simulink model "AECambioModoAutMan"  (R2020b)
settings: Solver=VariableStepAuto  StartTime=0.0  StopTime=50  RelTol=1e-3
settings Model: Creator=Juan  LastModifiedBy=Juan

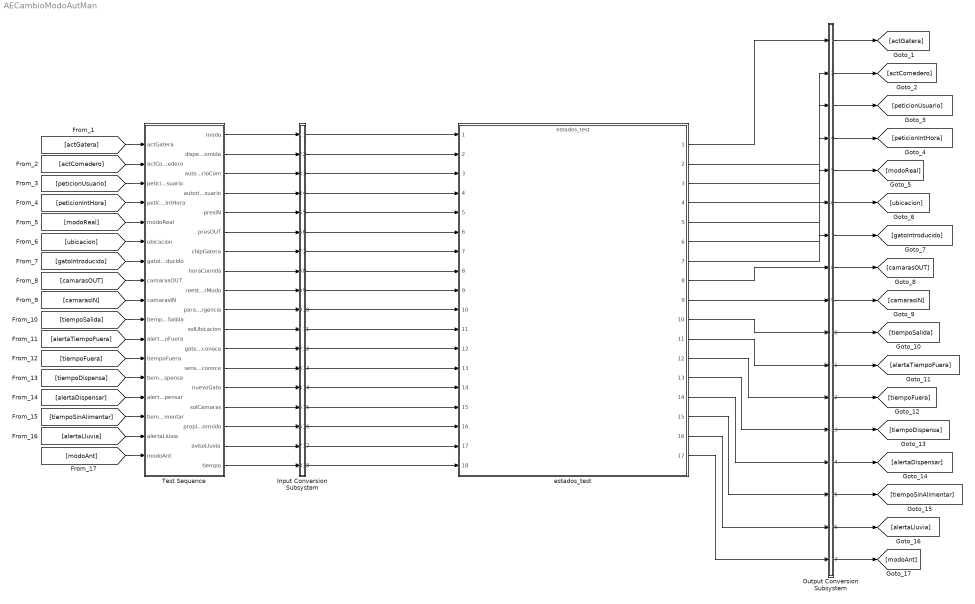
== system AECambioModoAutMan ==
  Input Conversion Subsystem : Subsystem  Tag=__SLT_ICS__  Description=|
      | Signal spec.
      | and routing
      settings: AttributesFormatString=%<Description>
  Output Conversion Subsystem : Subsystem  Tag=__SLT_OCS__  Description=|
      | Signal spec.
      | and routing
      settings: AttributesFormatString=%<Description>
  Test Sequence : Test Sequence  TreatAsAtomicUnit=on
  estados_test : ModelReference  ModelNameDialog=estados_test  SimulationMode=Normal  ModelReferenceVersion=2.162
  wires:
  Test Sequence/1(modo) -> Input Conversion Subsystem/1(Inport_1)
  Test Sequence/2(dispensaComida) -> Input Conversion Subsystem/2(Inport_2)
  Test Sequence/3(autorizUsuarioCom) -> Input Conversion Subsystem/3(Inport_3)
  Test Sequence/4(autorizUsuario) -> Input Conversion Subsystem/4(Inport_4)
  Test Sequence/5(presIN) -> Input Conversion Subsystem/5(Inport_5)
  Test Sequence/6(presOUT) -> Input Conversion Subsystem/6(Inport_6)
  Test Sequence/7(chipGatera) -> Input Conversion Subsystem/7(Inport_7)
  Test Sequence/8(horaComida) -> Input Conversion Subsystem/8(Inport_8)
  Test Sequence/9(reestablecerModo) -> Input Conversion Subsystem/9(Inport_9)
  Test Sequence/10(paradaEmergencia) -> Input Conversion Subsystem/10(Inport_10)
  Test Sequence/11(solUbicacion) -> Input Conversion Subsystem/11(Inport_11)
  Test Sequence/12(gateraReconoce) -> Input Conversion Subsystem/12(Inport_12)
  Test Sequence/13(sensorReconoce) -> Input Conversion Subsystem/13(Inport_13)
  Test Sequence/14(nuevoGato) -> Input Conversion Subsystem/14(Inport_14)
  Test Sequence/15(solCamaras) -> Input Conversion Subsystem/15(Inport_15)
  Test Sequence/16(propietarioDormido) -> Input Conversion Subsystem/16(Inport_16)
  Test Sequence/17(avisoLluvia) -> Input Conversion Subsystem/17(Inport_17)
  Test Sequence/18(tiempo) -> Input Conversion Subsystem/18(Inport_18)
  [actGatera] -> Test Sequence/1(actGatera)
  [actComedero] -> Test Sequence/2(actComedero)
  [peticionUsuario] -> Test Sequence/3(peticionUsuario)
  [peticionIntHora] -> Test Sequence/4(peticionIntHora)
  [modoReal] -> Test Sequence/5(modoReal)
  [ubicacion] -> Test Sequence/6(ubicacion)
  [gatoIntroducido] -> Test Sequence/7(gatoIntroducido)
  [camarasOUT] -> Test Sequence/8(camarasOUT)
  [camarasIN] -> Test Sequence/9(camarasIN)
  [tiempoSalida] -> Test Sequence/10(tiempoSalida)
  [alertaTiempoFuera] -> Test Sequence/11(alertaTiempoFuera)
  [tiempoFuera] -> Test Sequence/12(tiempoFuera)
  [tiempoDispensa] -> Test Sequence/13(tiempoDispensa)
  [alertaDispensar] -> Test Sequence/14(alertaDispensar)
  [tiempoSinAlimentar] -> Test Sequence/15(tiempoSinAlimentar)
  [alertaLluvia] -> Test Sequence/16(alertaLluvia)
  [modoAnt] -> Test Sequence/17(modoAnt)
  Output Conversion Subsystem/1(Outport_1) -> [actGatera]
  Output Conversion Subsystem/2(Outport_2) -> [actComedero]
  Output Conversion Subsystem/3(Outport_3) -> [peticionUsuario]
  Output Conversion Subsystem/4(Outport_4) -> [peticionIntHora]
  Output Conversion Subsystem/5(Outport_5) -> [modoReal]
  Output Conversion Subsystem/6(Outport_6) -> [ubicacion]
  Output Conversion Subsystem/7(Outport_7) -> [gatoIntroducido]
  Output Conversion Subsystem/8(Outport_8) -> [camarasOUT]
  Output Conversion Subsystem/9(Outport_9) -> [camarasIN]
  Output Conversion Subsystem/10(Outport_10) -> [tiempoSalida]
  Output Conversion Subsystem/11(Outport_11) -> [alertaTiempoFuera]
  Output Conversion Subsystem/12(Outport_12) -> [tiempoFuera]
  Output Conversion Subsystem/13(Outport_13) -> [tiempoDispensa]
  Output Conversion Subsystem/14(Outport_14) -> [alertaDispensar]
  Output Conversion Subsystem/15(Outport_15) -> [tiempoSinAlimentar]
  Output Conversion Subsystem/16(Outport_16) -> [alertaLluvia]
  Output Conversion Subsystem/17(Outport_17) -> [modoAnt]
  Input Conversion Subsystem/1(Outport_1) -> estados_test/1
  Input Conversion Subsystem/2(Outport_2) -> estados_test/2
  Input Conversion Subsystem/3(Outport_3) -> estados_test/3
  Input Conversion Subsystem/4(Outport_4) -> estados_test/4
  Input Conversion Subsystem/5(Outport_5) -> estados_test/5
  Input Conversion Subsystem/6(Outport_6) -> estados_test/6
  Input Conversion Subsystem/7(Outport_7) -> estados_test/7
  Input Conversion Subsystem/8(Outport_8) -> estados_test/8
  Input Conversion Subsystem/9(Outport_9) -> estados_test/9
  Input Conversion Subsystem/10(Outport_10) -> estados_test/10
  Input Conversion Subsystem/11(Outport_11) -> estados_test/11
  Input Conversion Subsystem/12(Outport_12) -> estados_test/12
  Input Conversion Subsystem/13(Outport_13) -> estados_test/13
  Input Conversion Subsystem/14(Outport_14) -> estados_test/14
  Input Conversion Subsystem/15(Outport_15) -> estados_test/15
  Input Conversion Subsystem/16(Outport_16) -> estados_test/16
  Input Conversion Subsystem/17(Outport_17) -> estados_test/17
  Input Conversion Subsystem/18(Outport_18) -> estados_test/18
  estados_test/1 -> Output Conversion Subsystem/1(Inport_1)
  estados_test/2 -> Output Conversion Subsystem/2(Inport_2)
  estados_test/3 -> Output Conversion Subsystem/3(Inport_3)
  estados_test/4 -> Output Conversion Subsystem/4(Inport_4)
  estados_test/5 -> Output Conversion Subsystem/5(Inport_5)
  estados_test/6 -> Output Conversion Subsystem/6(Inport_6)
  estados_test/7 -> Output Conversion Subsystem/7(Inport_7)
  estados_test/8 -> Output Conversion Subsystem/8(Inport_8)
  estados_test/9 -> Output Conversion Subsystem/9(Inport_9)
  estados_test/10 -> Output Conversion Subsystem/10(Inport_10)
  estados_test/11 -> Output Conversion Subsystem/11(Inport_11)
  estados_test/12 -> Output Conversion Subsystem/12(Inport_12)
  estados_test/13 -> Output Conversion Subsystem/13(Inport_13)
  estados_test/14 -> Output Conversion Subsystem/14(Inport_14)
  estados_test/15 -> Output Conversion Subsystem/15(Inport_15)
  estados_test/16 -> Output Conversion Subsystem/16(Inport_16)
  estados_test/17 -> Output Conversion Subsystem/17(Inport_17)

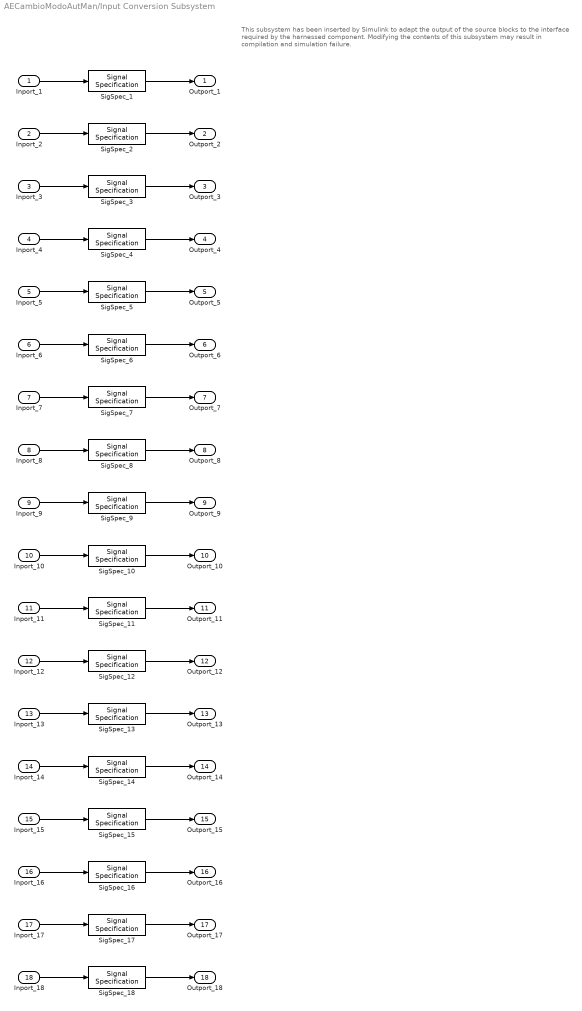
== system AECambioModoAutMan/Input Conversion Subsystem ==
  note: This subsystem has been inserted by Simulink to adapt the output of the source blocks to the interface required by the harnessed component.
      |  Modifying the contents of this subsystem may result in compilation and simulation failure.
  Inport_1 : Inport
  Inport_2 : Inport  Port=2
  Inport_3 : Inport  Port=3
  Inport_4 : Inport  Port=4
  Inport_5 : Inport  Port=5
  Inport_6 : Inport  Port=6
  Inport_7 : Inport  Port=7
  Inport_8 : Inport  Port=8
  Inport_9 : Inport  Port=9
  Inport_10 : Inport  Port=10
  Inport_11 : Inport  Port=11
  Inport_12 : Inport  Port=12
  Inport_13 : Inport  Port=13
  Inport_14 : Inport  Port=14
  Inport_15 : Inport  Port=15
  Inport_16 : Inport  Port=16
  Inport_17 : Inport  Port=17
  Inport_18 : Inport  Port=18
  SigSpec_{1..18} (18 alike) : SignalSpecification  OutDataTypeStr=double  Dimensions=[1]  SampleTime=[-1, 0]
  Outport_1 : Outport
  Outport_2 : Outport  Port=2
  Outport_3 : Outport  Port=3
  Outport_4 : Outport  Port=4
  Outport_5 : Outport  Port=5
  Outport_6 : Outport  Port=6
  Outport_7 : Outport  Port=7
  Outport_8 : Outport  Port=8
  Outport_9 : Outport  Port=9
  Outport_10 : Outport  Port=10
  Outport_11 : Outport  Port=11
  Outport_12 : Outport  Port=12
  Outport_13 : Outport  Port=13
  Outport_14 : Outport  Port=14
  Outport_15 : Outport  Port=15
  Outport_16 : Outport  Port=16
  Outport_17 : Outport  Port=17
  Outport_18 : Outport  Port=18
  wires:
  SigSpec_1/1 -> Outport_1/1
  Inport_1/1 -> SigSpec_1/1
  SigSpec_2/1 -> Outport_2/1
  Inport_2/1 -> SigSpec_2/1
  SigSpec_3/1 -> Outport_3/1
  Inport_3/1 -> SigSpec_3/1
  SigSpec_4/1 -> Outport_4/1
  Inport_4/1 -> SigSpec_4/1
  SigSpec_5/1 -> Outport_5/1
  Inport_5/1 -> SigSpec_5/1
  SigSpec_6/1 -> Outport_6/1
  Inport_6/1 -> SigSpec_6/1
  SigSpec_7/1 -> Outport_7/1
  Inport_7/1 -> SigSpec_7/1
  SigSpec_8/1 -> Outport_8/1
  Inport_8/1 -> SigSpec_8/1
  SigSpec_9/1 -> Outport_9/1
  Inport_9/1 -> SigSpec_9/1
  SigSpec_10/1 -> Outport_10/1
  Inport_10/1 -> SigSpec_10/1
  SigSpec_11/1 -> Outport_11/1
  Inport_11/1 -> SigSpec_11/1
  SigSpec_12/1 -> Outport_12/1
  Inport_12/1 -> SigSpec_12/1
  SigSpec_13/1 -> Outport_13/1
  Inport_13/1 -> SigSpec_13/1
  SigSpec_14/1 -> Outport_14/1
  Inport_14/1 -> SigSpec_14/1
  SigSpec_15/1 -> Outport_15/1
  Inport_15/1 -> SigSpec_15/1
  SigSpec_16/1 -> Outport_16/1
  Inport_16/1 -> SigSpec_16/1
  SigSpec_17/1 -> Outport_17/1
  Inport_17/1 -> SigSpec_17/1
  SigSpec_18/1 -> Outport_18/1
  Inport_18/1 -> SigSpec_18/1

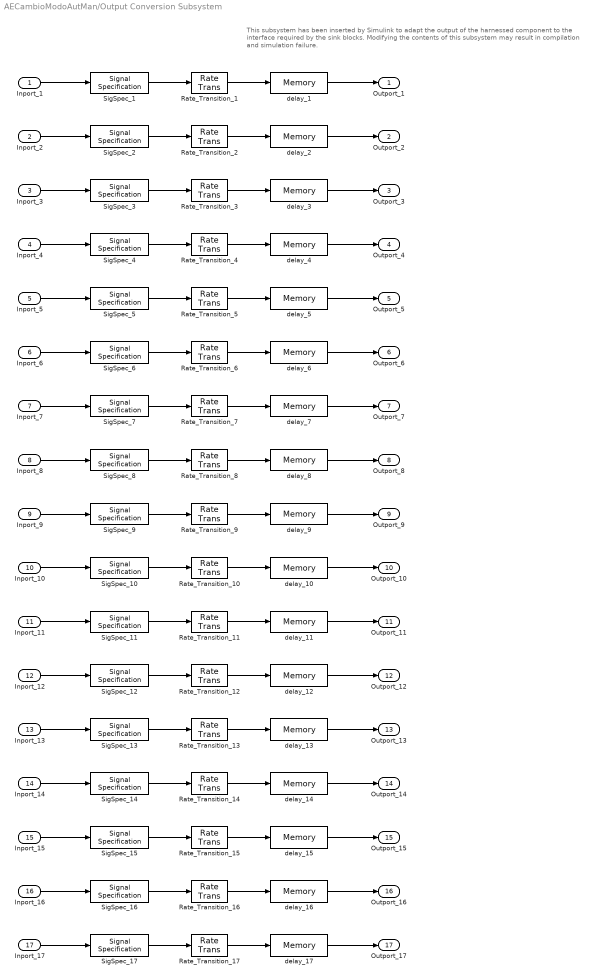
== system AECambioModoAutMan/Output Conversion Subsystem ==
  note: This subsystem has been inserted by Simulink to adapt the output of the harnessed component to the interface required by the sink blocks.
      |  Modifying the contents of this subsystem may result in compilation and simulation failure.
  Inport_1 : Inport
  Inport_2 : Inport  Port=2
  Inport_3 : Inport  Port=3
  Inport_4 : Inport  Port=4
  Inport_5 : Inport  Port=5
  Inport_6 : Inport  Port=6
  Inport_7 : Inport  Port=7
  Inport_8 : Inport  Port=8
  Inport_9 : Inport  Port=9
  Inport_10 : Inport  Port=10
  Inport_11 : Inport  Port=11
  Inport_12 : Inport  Port=12
  Inport_13 : Inport  Port=13
  Inport_14 : Inport  Port=14
  Inport_15 : Inport  Port=15
  Inport_16 : Inport  Port=16
  Inport_17 : Inport  Port=17
  Rate_Transition_{1..17} (17 alike) : RateTransition  OutPortSampleTimeOpt=Inherit
  SigSpec_{1..17} (17 alike) : SignalSpecification  OutDataTypeStr=double  Dimensions=[1]
  delay_{1..17} (17 alike) : Memory
  Outport_1 : Outport
  Outport_2 : Outport  Port=2
  Outport_3 : Outport  Port=3
  Outport_4 : Outport  Port=4
  Outport_5 : Outport  Port=5
  Outport_6 : Outport  Port=6
  Outport_7 : Outport  Port=7
  Outport_8 : Outport  Port=8
  Outport_9 : Outport  Port=9
  Outport_10 : Outport  Port=10
  Outport_11 : Outport  Port=11
  Outport_12 : Outport  Port=12
  Outport_13 : Outport  Port=13
  Outport_14 : Outport  Port=14
  Outport_15 : Outport  Port=15
  Outport_16 : Outport  Port=16
  Outport_17 : Outport  Port=17
  wires:
  Inport_1/1 -> SigSpec_1/1
  SigSpec_1/1 -> Rate_Transition_1/1
  Rate_Transition_1/1 -> delay_1/1
  delay_1/1 -> Outport_1/1
  Inport_2/1 -> SigSpec_2/1
  SigSpec_2/1 -> Rate_Transition_2/1
  Rate_Transition_2/1 -> delay_2/1
  delay_2/1 -> Outport_2/1
  Inport_3/1 -> SigSpec_3/1
  SigSpec_3/1 -> Rate_Transition_3/1
  Rate_Transition_3/1 -> delay_3/1
  delay_3/1 -> Outport_3/1
  Inport_4/1 -> SigSpec_4/1
  SigSpec_4/1 -> Rate_Transition_4/1
  Rate_Transition_4/1 -> delay_4/1
  delay_4/1 -> Outport_4/1
  Inport_5/1 -> SigSpec_5/1
  SigSpec_5/1 -> Rate_Transition_5/1
  Rate_Transition_5/1 -> delay_5/1
  delay_5/1 -> Outport_5/1
  Inport_6/1 -> SigSpec_6/1
  SigSpec_6/1 -> Rate_Transition_6/1
  Rate_Transition_6/1 -> delay_6/1
  delay_6/1 -> Outport_6/1
  Inport_7/1 -> SigSpec_7/1
  SigSpec_7/1 -> Rate_Transition_7/1
  Rate_Transition_7/1 -> delay_7/1
  delay_7/1 -> Outport_7/1
  Inport_8/1 -> SigSpec_8/1
  SigSpec_8/1 -> Rate_Transition_8/1
  Rate_Transition_8/1 -> delay_8/1
  delay_8/1 -> Outport_8/1
  Inport_9/1 -> SigSpec_9/1
  SigSpec_9/1 -> Rate_Transition_9/1
  Rate_Transition_9/1 -> delay_9/1
  delay_9/1 -> Outport_9/1
  Inport_10/1 -> SigSpec_10/1
  SigSpec_10/1 -> Rate_Transition_10/1
  Rate_Transition_10/1 -> delay_10/1
  delay_10/1 -> Outport_10/1
  Inport_11/1 -> SigSpec_11/1
  SigSpec_11/1 -> Rate_Transition_11/1
  Rate_Transition_11/1 -> delay_11/1
  delay_11/1 -> Outport_11/1
  Inport_12/1 -> SigSpec_12/1
  SigSpec_12/1 -> Rate_Transition_12/1
  Rate_Transition_12/1 -> delay_12/1
  delay_12/1 -> Outport_12/1
  Inport_13/1 -> SigSpec_13/1
  SigSpec_13/1 -> Rate_Transition_13/1
  Rate_Transition_13/1 -> delay_13/1
  delay_13/1 -> Outport_13/1
  Inport_14/1 -> SigSpec_14/1
  SigSpec_14/1 -> Rate_Transition_14/1
  Rate_Transition_14/1 -> delay_14/1
  delay_14/1 -> Outport_14/1
  Inport_15/1 -> SigSpec_15/1
  SigSpec_15/1 -> Rate_Transition_15/1
  Rate_Transition_15/1 -> delay_15/1
  delay_15/1 -> Outport_15/1
  Inport_16/1 -> SigSpec_16/1
  SigSpec_16/1 -> Rate_Transition_16/1
  Rate_Transition_16/1 -> delay_16/1
  delay_16/1 -> Outport_16/1
  Inport_17/1 -> SigSpec_17/1
  SigSpec_17/1 -> Rate_Transition_17/1
  Rate_Transition_17/1 -> delay_17/1
  delay_17/1 -> Outport_17/1

== stateflow chart AECambioModoAutMan/Test Sequence ==
  settings: stateMachineType=SIMPLIFIED_MACHINE
  state Run
    %% Initialize data outputs.
    modo = 0;
    dispensaComida = 0;
    autorizUsuarioCom = 0;
    autorizUsuario = 0;
    presIN = 0;
    presOUT = 0;
    chipGatera = 0;
    horaComida = 3;
    reestablecerModo = 0;
    paradaEmergencia = 0;
    solUbicacion = 0;
    gateraReconoce = 0;
    sensorReconoce = 0;
    nuevoGato = 0;
    solCamaras = 0;
    propietarioDormido = 0;
    avisoLluvia = 0;
    tiempo = 0;
  state step_1
    modo=1;
  (default) -> Run
  Run -> step_1 : [
      | after(10,sec)
      | ]
  data: actGatera input double size=[1]; actComedero input double size=[1]; peticionUsuario input double size=[1]; peticionIntHora input double size=[1]; modoReal input double size=[1]; ubicacion input double size=[1]; gatoIntroducido input double size=[1]; camarasOUT input double size=[1]; camarasIN input double size=[1]; tiempoSalida input double size=[1]; alertaTiempoFuera input double size=[1]; tiempoFuera input double size=[1]; tiempoDispensa input double size=[1]; alertaDispensar input double size=[1]; tiempoSinAlimentar input double size=[1]; alertaLluvia input double size=[1]; modoAnt input double size=[1]; modo output double size=[1]; dispensaComida output double size=[1]; autorizUsuarioCom output double size=[1]; autorizUsuario output double size=[1]; presIN output double size=[1]; presOUT output double size=[1]; chipGatera output double size=[1]; horaComida output double size=[1]; reestablecerModo output double size=[1]; paradaEmergencia output double size=[1]; solUbicacion output double size=[1]; gateraReconoce output double size=[1]; sensorReconoce output double size=[1]; nuevoGato output double size=[1]; solCamaras output double size=[1]; propietarioDormido output double size=[1]; avisoLluvia output double size=[1]; tiempo output double size=[1]
